simulink model "LQG_test"  (R2015a)
settings: Solver=ode5  StartTime=0.0  StopTime=160  FixedStep=5e-5  RelTol=1e-3
values from neighbouring files (symbols this model uses):
  Ak = [-672.634870495 -2626.58972998 -46.1193303275 25.5793500122 108.891317034 -102.718752792 -245.794654799 -577.315326704 39.8827087547 153.58157137 60.36854216 -207.81122515 ... (144 elements, 12x12)]    [controller_reduced.mat]    (also in main_matlab.m = rlqg.A)
  Bk = [0.204306341627 1.11161335273 -0.324978673641 2.85402340631 -4.5813117605 2.97328839236 -0.174709893359 1.31662160979 2.94898293865 13.5567055967 -0.791381118401 0.0552385579013]    [controller_reduced.mat]    (also in main_matlab.m = rlqg.B)
  Ck = [534.788956442 909.016401092 107.069958755 -410.092366717 -1097.26369634 478.53061829 -894.210554118 460.341899649 -450.064931583 371.993181033 532.787728171 55.8162878584 ... (24 elements, 2x12)]    [controller_reduced.mat]    (also in main_matlab.m = rlqg.C)
  Dk = [0 0]    [controller_reduced.mat]    (also in main_matlab.m = rlqg.D)
undefined symbols (not defined in the file or in its folder): Af, Bf, Cf, Hf
libraries: simulink x1
settings Model: Creator=p4wp4w  LastModifiedBy=Ablah

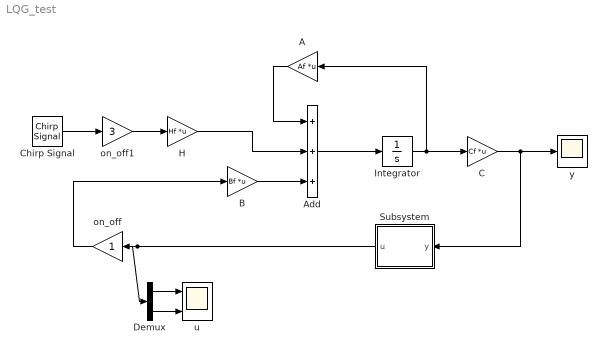
== system LQG_test ==
  A : Gain  Gain=Af  Multiplication=Matrix(K*u)
  Add : Sum  Inputs=+++
  B : Gain  Gain=Bf  Multiplication=Matrix(K*u)
  C : Gain  Gain=Cf  Multiplication=Matrix(K*u)
  Chirp Signal : simulink/Sources/Chirp Signal  f1=0.1  T=80  f2=800
  Demux : Demux  Outputs=2
  H : Gain  Gain=Hf  Multiplication=Matrix(K*u)
  Integrator : Integrator
  Subsystem : Subsystem
  on_off : Gain
  on_off1 : Gain  Gain=3
  u : Scope  NumInputPorts=2
      settings: YMin=-5~-5  YMax=5~5
  y : Scope
      settings: YMin=-0.03  YMax=0.03
  wires:
  Add/1 -> Integrator/1
  A/1 -> Add/1
  B/1 -> Add/3
  Integrator/1 -> C/1, A/1
  H/1 -> Add/2
  Chirp Signal/1 -> on_off1/1
  on_off/1 -> B/1
  Demux/1 -> u/1
  Demux/2 -> u/2
  C/1 -> Subsystem/1(y), y/1
  Subsystem/1("u ") -> Demux/1, on_off/1
  on_off1/1 -> H/1

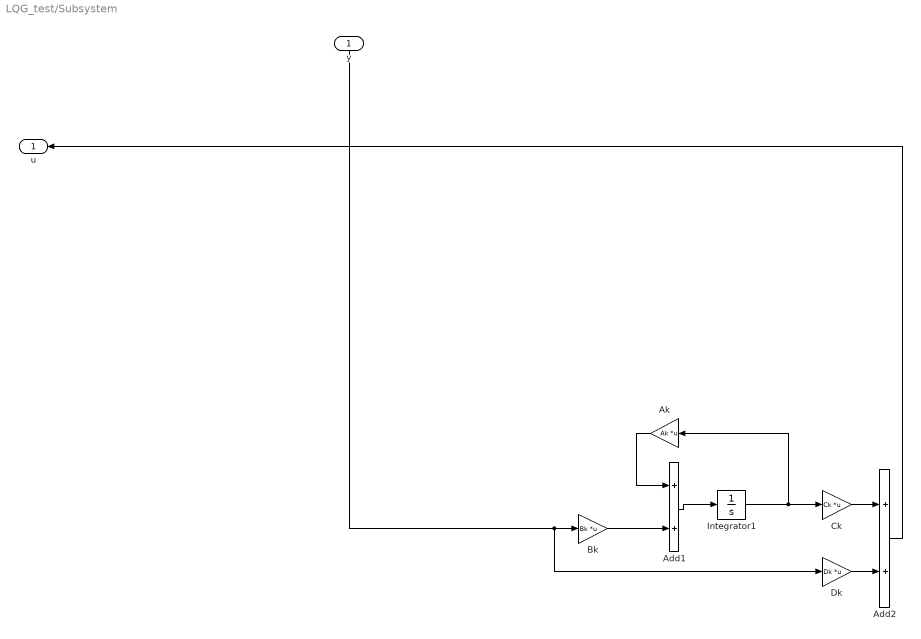
== system LQG_test/Subsystem ==
  y : Inport
  Add1 : Sum
  Add2 : Sum
  Ak : Gain  Gain=Ak  Multiplication=Matrix(K*u)
  Bk : Gain  Gain=Bk  Multiplication=Matrix(K*u)
  Ck : Gain  Gain=Ck  Multiplication=Matrix(K*u)
  Dk : Gain  Gain=Dk  Multiplication=Matrix(K*u)
  Integrator1 : Integrator
  "u " : Outport
  wires:
  y/1 -> Bk/1, Dk/1
  Add2/1 -> "u "/1
  Bk/1 -> Add1/2
  Ak/1 -> Add1/1
  Add1/1 -> Integrator1/1
  Dk/1 -> Add2/2
  Integrator1/1 -> Ck/1, Ak/1
  Ck/1 -> Add2/1
